simulink model "sys_ctrl_obs_luenberger_int_theta"  (Simulink 7.9)
settings: Solver=ode45  StartTime=0.0  StopTime=Tt  FixedStep=0.002  RelTol=1e-3
undefined symbols (not defined in the file): a, A11, A12, A21, A22, alpha_max, alpha_min, b, B1, B2, c, dalpha_max, dalpha_min, dtheta_max, dtheta_min, K, Knoise, L, theta_max, theta_min, Ts, x_0
libraries: simulink x1
settings Model: Creator=pdoren  LastModifiedBy=matias  CovModelRefEnable=off
settings SolverCC: ZeroCrossAlgorithm=Adaptive
settings DataIOCC: SaveFormat=StructureWithTime  SignalLoggingSaveFormat=Dataset
settings OptimizationCC: ExpressionDepthLimit=128  EfficientMapNaN2IntZero=off
settings DebuggingCC: ConsistencyChecking=warning  UnderspecifiedInitializationDetection=Simplified  MergeDetectMultiDrivingBlocksExec=error  TimeAdjustmentMsg=warning
settings HardwareCC: ProdBitPerPointer=64  ProdLargestAtomicFloat=Float  ProdIntDivRoundTo=Zero  ProdEndianess=LittleEndian  ProdHWDeviceType=Specified
settings CodeAppCC: CustomSymbolStrType=$N$R$M_T
settings GRTTargetCC: CodeReplacementLibrary=C89/C90 (ANSI)  GeneratePreprocessorConditionals=Use local settings  CombineOutputUpdateFcns=off  GRTInterface=on

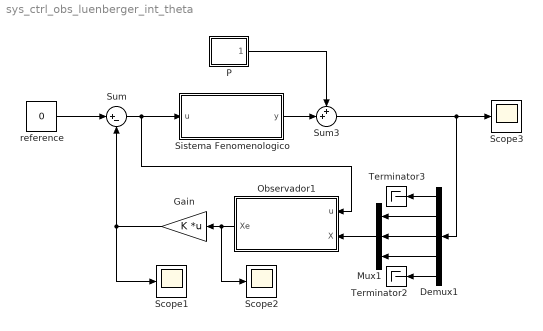
== system sys_ctrl_obs_luenberger_int_theta ==
  Demux1 : Demux  Outputs=5
  Gain : Gain  Gain=K  Multiplication=Matrix(K*u)
  Mux1 : Mux  Inputs=3
  Observador1 : Subsystem
  P : Subsystem
  Scope1 : Scope
      settings: YMin=-16.24296  YMax=1.5745  SaveName=Vin
  Scope2 : Scope
      settings: YMin=-0.92194  YMax=2.92896  SaveName=states_feno_obs
  Scope3 : Scope
      settings: YMin=-0.8209  YMax=2.93262  SaveName=states_feno
  Sistema Fenomenologico : Subsystem
  Sum : Sum  Inputs=|+-
  Sum3 : Sum  Inputs=++|
  Terminator2 : Terminator
  Terminator3 : Terminator
  reference : Constant  Value=0
  wires:
  Sum/1 -> Sistema Fenomenologico/1(u), Observador1/1(u)
  Sistema Fenomenologico/1(y) -> Sum3/2
  reference/1 -> Sum/1
  P/1(Out1) -> Sum3/1
  Gain/1 -> Sum/2, Scope1/1
  Demux1/2 -> Mux1/1
  Demux1/3 -> Mux1/2
  Demux1/4 -> Mux1/3
  Demux1/1 -> Terminator3/1
  Demux1/5 -> Terminator2/1
  Mux1/1 -> Observador1/2(X)
  Observador1/1(Xe) -> Gain/1, Scope2/1
  Sum3/1 -> Scope3/1, Demux1/1

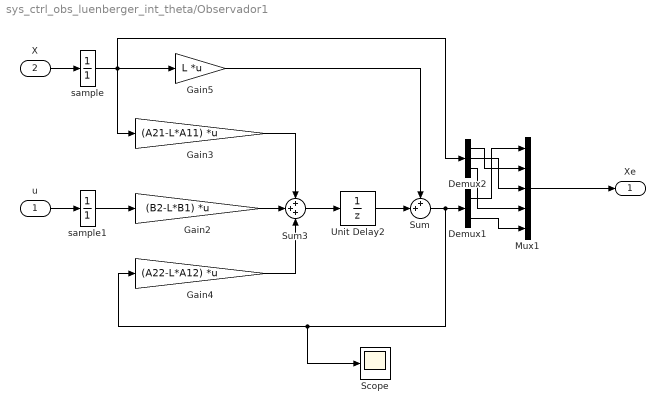
== system sys_ctrl_obs_luenberger_int_theta/Observador1 ==
  u : Inport
  X : Inport  Port=2
  Demux1 : Demux  Outputs=2
  Demux2 : Demux  Outputs=3
  Gain2 : Gain  Gain=(B2-L*B1)  Multiplication=Matrix(K*u)
  Gain3 : Gain  Gain=(A21-L*A11)  Multiplication=Matrix(K*u)
  Gain4 : Gain  Gain=(A22-L*A12)  Multiplication=Matrix(K*u)
  Gain5 : Gain  Gain=L  Multiplication=Matrix(K*u)
  Mux1 : Mux  Inputs=5
  Scope : Scope
      settings: YMin=-37139.72476  YMax=4126.63608
  Sum : Sum  Inputs=++|
  Sum3 : Sum  Inputs=+++
  Unit Delay2 : UnitDelay  SampleTime=Ts
  sample : DiscreteTransferFcn  Denominator=[1]  SampleTime=Ts
  sample1 : DiscreteTransferFcn  Denominator=[1]  SampleTime=Ts
  Xe : Outport
  wires:
  Gain3/1 -> Sum3/1
  Gain4/1 -> Sum3/3
  Unit Delay2/1 -> Sum/2
  Sum3/1 -> Unit Delay2/1
  Gain2/1 -> Sum3/2
  Sum/1 -> Scope/1, Gain4/1, Demux1/1
  Gain5/1 -> Sum/1
  Demux2/2 -> Mux1/3
  Demux2/1 -> Mux1/2
  Demux1/1 -> Mux1/1
  Mux1/1 -> Xe/1
  Demux2/3 -> Mux1/4
  Demux1/2 -> Mux1/5
  X/1 -> sample/1
  u/1 -> sample1/1
  sample/1 -> Gain3/1, Demux2/1, Gain5/1
  sample1/1 -> Gain2/1

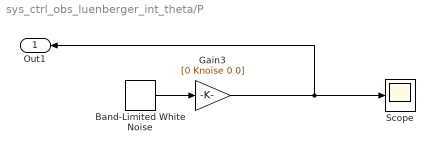
== system sys_ctrl_obs_luenberger_int_theta/P ==
  Band-Limited White Noise : simulink/Sources/Band-Limited White Noise  Cov=[0.01]  Ts=0.002  seed=[23341]
  Gain3 : Gain  Gain=[0 Knoise 0 0]
  Scope : Scope
      settings: YMin=-0.0000028  YMax=0.0000062
  Out1 : Outport
  wires:
  Gain3/1 -> Out1/1, Scope/1
  Band-Limited White Noise/1 -> Gain3/1

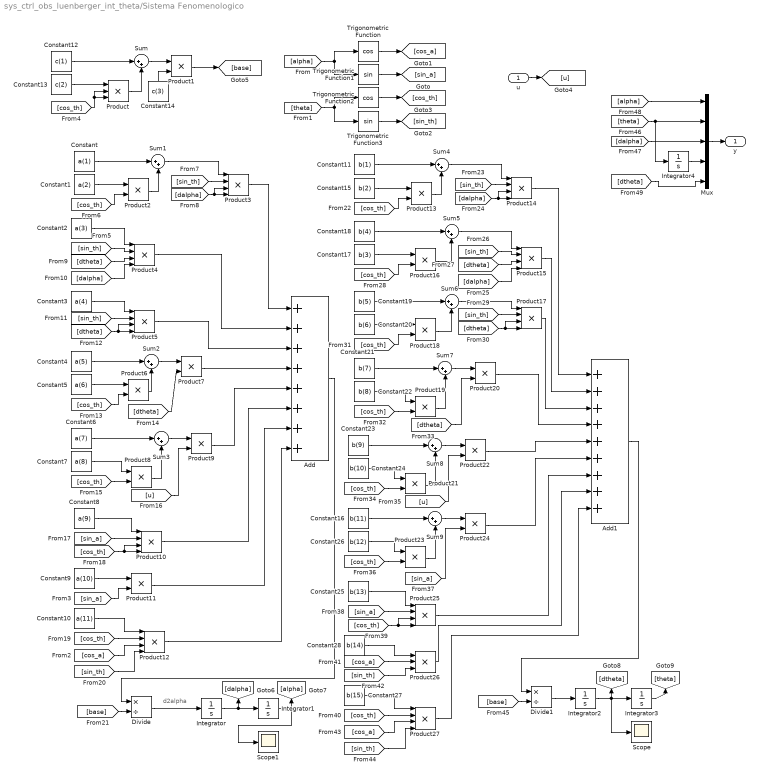
== system sys_ctrl_obs_luenberger_int_theta/Sistema Fenomenologico ==
  note: d2alpha
  u : Inport
  Add : Sum  Inputs=++++++++
  Add1 : Sum  Inputs=+++++++++
  Constant : Constant  Value=a(1)
  Constant1 : Constant  Value=a(2)
  Constant10 : Constant  Value=a(11)
  Constant11 : Constant  Value=b(1)
  Constant12 : Constant  Value=c(1)
  Constant13 : Constant  Value=c(2)
  Constant14 : Constant  Value=c(3)
  Constant15 : Constant  Value=b(2)
  Constant16 : Constant  Value=b(11)
  Constant17 : Constant  Value=b(3)
  Constant18 : Constant  Value=b(4)
  Constant19 : Constant  Value=b(5)
  Constant2 : Constant  Value=a(3)
  Constant20 : Constant  Value=b(6)
  Constant21 : Constant  Value=b(7)
  Constant22 : Constant  Value=b(8)
  Constant23 : Constant  Value=b(9)
  Constant24 : Constant  Value=b(10)
  Constant25 : Constant  Value=b(13)
  Constant26 : Constant  Value=b(12)
  Constant27 : Constant  Value=b(15)
  Constant28 : Constant  Value=b(14)
  Constant3 : Constant  Value=a(4)
  Constant4 : Constant  Value=a(5)
  Constant5 : Constant  Value=a(6)
  Constant6 : Constant  Value=a(7)
  Constant7 : Constant  Value=a(8)
  Constant8 : Constant  Value=a(9)
  Constant9 : Constant  Value=a(10)
  Divide : Product  Inputs=*/
  Divide1 : Product  Inputs=*/
  Integrator : Integrator  InitialCondition=x_0(3)  UpperSaturationLimit=dalpha_max  LowerSaturationLimit=dalpha_min
  Integrator1 : Integrator  InitialCondition=x_0(1)  UpperSaturationLimit=alpha_max  LowerSaturationLimit=alpha_min
  Integrator2 : Integrator  InitialCondition=x_0(5)  UpperSaturationLimit=dtheta_max  LowerSaturationLimit=dtheta_min
  Integrator3 : Integrator  InitialCondition=x_0(2)  UpperSaturationLimit=theta_max  LowerSaturationLimit=theta_min
  Integrator4 : Integrator
  Mux : Mux  Inputs=5
  Product : Product  Inputs=3  RndMeth=Zero
  Product{1..2,6..9,11,13,16,18..24} (16 alike) : Product  RndMeth=Zero
  Product{3..5,10,12,14..15,17,25,27} (10 alike) : Product  Inputs=4  RndMeth=Zero
  Product26 : Product  Inputs=3  RndMeth=Zero
  Scope : Scope
      settings: YMin=-52646.18239  YMax=473815.64154  SaveName=dtheta
  Scope1 : Scope
      settings: YMin=-5.37162  YMax=0.77142  SaveName=alpha
  Sum{,1..9} (10 alike) : Sum  Inputs=|++
  Trigonometric Function : Trigonometry  Operator=cos
  Trigonometric Function1 : Trigonometry
  Trigonometric Function2 : Trigonometry  Operator=cos
  Trigonometric Function3 : Trigonometry
  y : Outport
  wires:
  [alpha] -> Trigonometric Function/1, Trigonometric Function1/1
  [theta] -> Trigonometric Function2/1, Trigonometric Function3/1
  Trigonometric Function1/1 -> [sin_a]
  Trigonometric Function/1 -> [cos_a]
  Trigonometric Function2/1 -> [cos_th]
  Trigonometric Function3/1 -> [sin_th]
  Constant12/1 -> Sum/1
  Product/1 -> Sum/2
  Constant13/1 -> Product/1
  [cos_th] -> Product/2, Product/3
  Sum/1 -> Product1/1
  Constant14/1 -> Product1/2
  Constant/1 -> Sum1/1
  Constant1/1 -> Product2/1
  [cos_th] -> Product2/2
  Product2/1 -> Sum1/2
  Sum1/1 -> Product3/1
  [sin_th] -> Product3/2
  [dalpha] -> Product3/3, Product3/4
  Constant2/1 -> Product4/1
  [sin_th] -> Product4/2
  [dalpha] -> Product4/4
  [dtheta] -> Product4/3
  Constant3/1 -> Product5/1
  [sin_th] -> Product5/2
  [dtheta] -> Product5/3, Product5/4
  Constant4/1 -> Sum2/1
  Constant5/1 -> Product6/1
  Product6/1 -> Sum2/2
  [cos_th] -> Product6/2
  Sum2/1 -> Product7/1
  [dtheta] -> Product7/2
  Constant6/1 -> Sum3/1
  Constant7/1 -> Product8/1
  [cos_th] -> Product8/2
  Product8/1 -> Sum3/2
  Sum3/1 -> Product9/1
  [u] -> Product9/2
  u/1 -> [u]
  Constant8/1 -> Product10/1
  [sin_a] -> Product10/2
  [cos_th] -> Product10/3, Product10/4
  Constant9/1 -> Product11/1
  [sin_a] -> Product11/2
  Constant10/1 -> Product12/1
  [cos_th] -> Product12/2
  [cos_a] -> Product12/3
  [sin_th] -> Product12/4
  Product3/1 -> Add/1
  Product4/1 -> Add/2
  Product5/1 -> Add/3
  Product7/1 -> Add/4
  Product9/1 -> Add/5
  Product10/1 -> Add/6
  Product11/1 -> Add/7
  Product12/1 -> Add/8
  Product1/1 -> [base]
  [base] -> Divide/2
  Integrator/1 -> Integrator1/1, [dalpha]
  Integrator1/1 -> Scope1/1, [alpha]
  Divide/1 -> Integrator/1
  Add/1 -> Divide/1
  Constant11/1 -> Sum4/1
  Constant15/1 -> Product13/1
  [cos_th] -> Product13/2
  Product13/1 -> Sum4/2
  Sum4/1 -> Product14/1
  [sin_th] -> Product14/2
  [dalpha] -> Product14/3, Product14/4
  [sin_th] -> Product15/2
  [dalpha] -> Product15/4
  [dtheta] -> Product15/3
  Constant17/1 -> Product16/1
  [cos_th] -> Product16/2
  Constant18/1 -> Sum5/1
  Product16/1 -> Sum5/2
  Sum5/1 -> Product15/1
  [sin_th] -> Product17/2
  [dtheta] -> Product17/3, Product17/4
  Constant20/1 -> Product18/1
  [cos_th] -> Product18/2
  Constant19/1 -> Sum6/1
  Product18/1 -> Sum6/2
  Sum6/1 -> Product17/1
  Constant21/1 -> Sum7/1
  Constant22/1 -> Product19/1
  [cos_th] -> Product19/2
  Product19/1 -> Sum7/2
  Sum7/1 -> Product20/1
  [dtheta] -> Product20/2
  Constant23/1 -> Sum8/1
  Constant24/1 -> Product21/1
  [cos_th] -> Product21/2
  Product21/1 -> Sum8/2
  Sum8/1 -> Product22/1
  [u] -> Product22/2
  Constant16/1 -> Sum9/1
  Constant26/1 -> Product23/1
  [cos_th] -> Product23/2
  Product23/1 -> Sum9/2
  Sum9/1 -> Product24/1
  [sin_a] -> Product24/2
  Constant25/1 -> Product25/1
  [sin_a] -> Product25/2
  [cos_th] -> Product25/3, Product25/4
  Constant28/1 -> Product26/1
  [sin_th] -> Product26/3
  [cos_a] -> Product26/2
  Constant27/1 -> Product27/1
  [cos_th] -> Product27/2
  [cos_a] -> Product27/3
  [sin_th] -> Product27/4
  Product14/1 -> Add1/1
  Product15/1 -> Add1/2
  Product17/1 -> Add1/3
  Product20/1 -> Add1/4
  Product22/1 -> Add1/5
  Product24/1 -> Add1/6
  Product25/1 -> Add1/7
  Product26/1 -> Add1/8
  Product27/1 -> Add1/9
  [base] -> Divide1/2
  Integrator2/1 -> Scope/1, Integrator3/1, [dtheta]
  Integrator3/1 -> [theta]
  Divide1/1 -> Integrator2/1
  Add1/1 -> Divide1/1
  Mux/1 -> y/1
  [theta] -> Mux/2, Integrator4/1
  [dalpha] -> Mux/3
  [alpha] -> Mux/1
  [dtheta] -> Mux/5
  Integrator4/1 -> Mux/4
